simulink library "pack_105s34p_structured"  (R2023b)
settings: Solver=VariableStepAuto  StartTime=0.0  StopTime=10.0  RelTol=1e-3
undefined symbols (not defined in the file): battery_builder_rtmsupport, gcbh
libraries: pack_105s34p_structured_lib x156
(part 3 of 7)

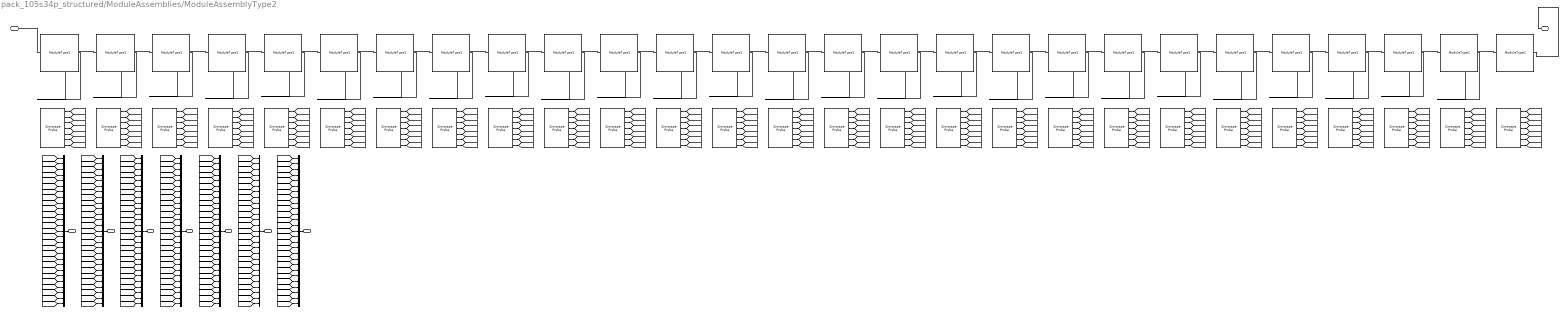
== system pack_105s34p_structured/ModuleAssemblies/ModuleAssemblyType2 ==
  note: Battery Modules
  note: Output Signals
  Module01 : pack_105s34p_structured_lib/Modules/ModuleType1  SOC_vecCell=[0, .1, .25, .5, .75, .9, 1]  T_vecCell=[278, 293, 313] K  V0_matCell=[3.49, 3.5, 3.51; 3.55, 3.57, 3.56; 3.62, 3.63, 3.64; 3.71, 3.71, 3.72; 3.91, 3.93, 3.94; 4.07, 4.08, 4.08; 4.19, 4.19, 4.19] V  V_rangeCell=[0, inf] V  R0_matCell=[.0117, .0085, .009; .011, .0085, .009; .0114, .0087, .0092; .0107, .0082, .0088; .0107, .0083, .0091; .0113, .0085, .0089; .0116, .0085, .0089] Ohm  AHCell=27 A*hr  extrapolation_optionCell=simscape.enum.extrapolation.nearest  R1_matCell=[.0109, .0029, .0013; .0069, .0024, .0012; .0047, .0026, .0013; .0034, .0016, .001; .0033, .0023, .0014; .0033, .0018, .0011; .0028, .0017, .0011] Ohm  tau1_matCell=[20, 36, 39; 31, 45, 39; 109, 105, 61; 36, 29, 26; 59, 77, 67; 40, 33, 29; 25, 39, 33] s  R2_matCell=[.0109, .0029, .0013; .0069, .0024, .0012; .0047, .0026, .0013; .0034, .0016, .001; .0033, .0023, .0014; .0033, .0018, .0011; .0028, .0017, .0011] Ohm  tau2_matCell=[20, 36, 39; 31, 45, 39; 109, 105, 61; 36, 29, 26; 59, 77, 67; 40, 33, 29; 25, 39, 33] s  R3_matCell=[.0109, .0029, .0013; .0069, .0024, .0012; .0047, .0026, .0013; .0034, .0016, .001; .0033, .0023, .0014; .0033, .0018, .0011; .0028, .0017, .0011] Ohm  tau3_matCell=[20, 36, 39; 31, 45, 39; 109, 105, 61; 36, 29, 26; 59, 77, 67; 40, 33, 29; 25, 39, 33] s  thermal_massCell=100 J/K  P=34  S=1  iCell_specify=off  iCell_priority=None  iCell=0 A  iCell_nominal_specify=off  iCell_nominal_unit=A  iCell_nominal_value=1  vCell_specify=off  vCell_priority=None  vCell=0 V  vCell_nominal_specify=off  vCell_nominal_unit=V  vCell_nominal_value=1  socCell_specify=off  socCell_priority=High  socCell=1  socCell_nominal_specify=off  socCell_nominal_unit=1  socCell_nominal_value=1  numCyclesCell_specify=off  numCyclesCell_priority=High  numCyclesCell=0  numCyclesCell_nominal_specify=off  numCyclesCell_nominal_unit=1  numCyclesCell_nominal_value=1  temperatureCell_specify=off  temperatureCell_priority=High  temperatureCell=298.15 K  temperatureCell_nominal_specify=off  temperatureCell_nominal_unit=K  temperatureCell_nominal_value=1  vParallelAssembly_specify=off  vParallelAssembly_priority=None  vParallelAssembly=0 V  vParallelAssembly_nominal_specify=off  vParallelAssembly_nominal_unit=V  vParallelAssembly_nominal_value=1  socParallelAssembly_specify=off  socParallelAssembly_priority=None  socParallelAssembly=1  socParallelAssembly_nominal_specify=off  socParallelAssembly_nominal_unit=1  socParallelAssembly_nominal_value=1
      settings: InternalSimscapePortConfiguration="{\"Bottom\":[{\"id\":\"n\",\"label\":\"-\",\"type\":\"foundation.electrical.electrical\"}],\"Left\":[],\"Right\":[],\"Top\":[{\"id\":\"p\",\"label\":\"+\",\"type\":\"foundation.electrical.electrical\"}]}"
  Module01_outputs : SimscapeProbe  BoundBlock=406  Variables={iCell, numCyclesCell, socCell, socParallelAssembly, temperatureCell, vCell, vParallelAssembly}
  Module02 : pack_105s34p_structured_lib/Modules/ModuleType1  SOC_vecCell=[0, .1, .25, .5, .75, .9, 1]  T_vecCell=[278, 293, 313] K  V0_matCell=[3.49, 3.5, 3.51; 3.55, 3.57, 3.56; 3.62, 3.63, 3.64; 3.71, 3.71, 3.72; 3.91, 3.93, 3.94; 4.07, 4.08, 4.08; 4.19, 4.19, 4.19] V  V_rangeCell=[0, inf] V  R0_matCell=[.0117, .0085, .009; .011, .0085, .009; .0114, .0087, .0092; .0107, .0082, .0088; .0107, .0083, .0091; .0113, .0085, .0089; .0116, .0085, .0089] Ohm  AHCell=27 A*hr  extrapolation_optionCell=simscape.enum.extrapolation.nearest  R1_matCell=[.0109, .0029, .0013; .0069, .0024, .0012; .0047, .0026, .0013; .0034, .0016, .001; .0033, .0023, .0014; .0033, .0018, .0011; .0028, .0017, .0011] Ohm  tau1_matCell=[20, 36, 39; 31, 45, 39; 109, 105, 61; 36, 29, 26; 59, 77, 67; 40, 33, 29; 25, 39, 33] s  R2_matCell=[.0109, .0029, .0013; .0069, .0024, .0012; .0047, .0026, .0013; .0034, .0016, .001; .0033, .0023, .0014; .0033, .0018, .0011; .0028, .0017, .0011] Ohm  tau2_matCell=[20, 36, 39; 31, 45, 39; 109, 105, 61; 36, 29, 26; 59, 77, 67; 40, 33, 29; 25, 39, 33] s  R3_matCell=[.0109, .0029, .0013; .0069, .0024, .0012; .0047, .0026, .0013; .0034, .0016, .001; .0033, .0023, .0014; .0033, .0018, .0011; .0028, .0017, .0011] Ohm  tau3_matCell=[20, 36, 39; 31, 45, 39; 109, 105, 61; 36, 29, 26; 59, 77, 67; 40, 33, 29; 25, 39, 33] s  thermal_massCell=100 J/K  P=34  S=1  iCell_specify=off  iCell_priority=None  iCell=0 A  iCell_nominal_specify=off  iCell_nominal_unit=A  iCell_nominal_value=1  vCell_specify=off  vCell_priority=None  vCell=0 V  vCell_nominal_specify=off  vCell_nominal_unit=V  vCell_nominal_value=1  socCell_specify=off  socCell_priority=High  socCell=1  socCell_nominal_specify=off  socCell_nominal_unit=1  socCell_nominal_value=1  numCyclesCell_specify=off  numCyclesCell_priority=High  numCyclesCell=0  numCyclesCell_nominal_specify=off  numCyclesCell_nominal_unit=1  numCyclesCell_nominal_value=1  temperatureCell_specify=off  temperatureCell_priority=High  temperatureCell=298.15 K  temperatureCell_nominal_specify=off  temperatureCell_nominal_unit=K  temperatureCell_nominal_value=1  vParallelAssembly_specify=off  vParallelAssembly_priority=None  vParallelAssembly=0 V  vParallelAssembly_nominal_specify=off  vParallelAssembly_nominal_unit=V  vParallelAssembly_nominal_value=1  socParallelAssembly_specify=off  socParallelAssembly_priority=None  socParallelAssembly=1  socParallelAssembly_nominal_specify=off  socParallelAssembly_nominal_unit=1  socParallelAssembly_nominal_value=1
      settings: InternalSimscapePortConfiguration="{\"Bottom\":[{\"id\":\"n\",\"label\":\"-\",\"type\":\"foundation.electrical.electrical\"}],\"Left\":[],\"Right\":[],\"Top\":[{\"id\":\"p\",\"label\":\"+\",\"type\":\"foundation.electrical.electrical\"}]}"
  Module02_outputs : SimscapeProbe  BoundBlock=407  Variables={iCell, numCyclesCell, socCell, socParallelAssembly, temperatureCell, vCell, vParallelAssembly}
  Module03 : pack_105s34p_structured_lib/Modules/ModuleType1  SOC_vecCell=[0, .1, .25, .5, .75, .9, 1]  T_vecCell=[278, 293, 313] K  V0_matCell=[3.49, 3.5, 3.51; 3.55, 3.57, 3.56; 3.62, 3.63, 3.64; 3.71, 3.71, 3.72; 3.91, 3.93, 3.94; 4.07, 4.08, 4.08; 4.19, 4.19, 4.19] V  V_rangeCell=[0, inf] V  R0_matCell=[.0117, .0085, .009; .011, .0085, .009; .0114, .0087, .0092; .0107, .0082, .0088; .0107, .0083, .0091; .0113, .0085, .0089; .0116, .0085, .0089] Ohm  AHCell=27 A*hr  extrapolation_optionCell=simscape.enum.extrapolation.nearest  R1_matCell=[.0109, .0029, .0013; .0069, .0024, .0012; .0047, .0026, .0013; .0034, .0016, .001; .0033, .0023, .0014; .0033, .0018, .0011; .0028, .0017, .0011] Ohm  tau1_matCell=[20, 36, 39; 31, 45, 39; 109, 105, 61; 36, 29, 26; 59, 77, 67; 40, 33, 29; 25, 39, 33] s  R2_matCell=[.0109, .0029, .0013; .0069, .0024, .0012; .0047, .0026, .0013; .0034, .0016, .001; .0033, .0023, .0014; .0033, .0018, .0011; .0028, .0017, .0011] Ohm  tau2_matCell=[20, 36, 39; 31, 45, 39; 109, 105, 61; 36, 29, 26; 59, 77, 67; 40, 33, 29; 25, 39, 33] s  R3_matCell=[.0109, .0029, .0013; .0069, .0024, .0012; .0047, .0026, .0013; .0034, .0016, .001; .0033, .0023, .0014; .0033, .0018, .0011; .0028, .0017, .0011] Ohm  tau3_matCell=[20, 36, 39; 31, 45, 39; 109, 105, 61; 36, 29, 26; 59, 77, 67; 40, 33, 29; 25, 39, 33] s  thermal_massCell=100 J/K  P=34  S=1  iCell_specify=off  iCell_priority=None  iCell=0 A  iCell_nominal_specify=off  iCell_nominal_unit=A  iCell_nominal_value=1  vCell_specify=off  vCell_priority=None  vCell=0 V  vCell_nominal_specify=off  vCell_nominal_unit=V  vCell_nominal_value=1  socCell_specify=off  socCell_priority=High  socCell=1  socCell_nominal_specify=off  socCell_nominal_unit=1  socCell_nominal_value=1  numCyclesCell_specify=off  numCyclesCell_priority=High  numCyclesCell=0  numCyclesCell_nominal_specify=off  numCyclesCell_nominal_unit=1  numCyclesCell_nominal_value=1  temperatureCell_specify=off  temperatureCell_priority=High  temperatureCell=298.15 K  temperatureCell_nominal_specify=off  temperatureCell_nominal_unit=K  temperatureCell_nominal_value=1  vParallelAssembly_specify=off  vParallelAssembly_priority=None  vParallelAssembly=0 V  vParallelAssembly_nominal_specify=off  vParallelAssembly_nominal_unit=V  vParallelAssembly_nominal_value=1  socParallelAssembly_specify=off  socParallelAssembly_priority=None  socParallelAssembly=1  socParallelAssembly_nominal_specify=off  socParallelAssembly_nominal_unit=1  socParallelAssembly_nominal_value=1
      settings: InternalSimscapePortConfiguration="{\"Bottom\":[{\"id\":\"n\",\"label\":\"-\",\"type\":\"foundation.electrical.electrical\"}],\"Left\":[],\"Right\":[],\"Top\":[{\"id\":\"p\",\"label\":\"+\",\"type\":\"foundation.electrical.electrical\"}]}"
  Module03_outputs : SimscapeProbe  BoundBlock=408  Variables={iCell, numCyclesCell, socCell, socParallelAssembly, temperatureCell, vCell, vParallelAssembly}
  Module04 : pack_105s34p_structured_lib/Modules/ModuleType1  SOC_vecCell=[0, .1, .25, .5, .75, .9, 1]  T_vecCell=[278, 293, 313] K  V0_matCell=[3.49, 3.5, 3.51; 3.55, 3.57, 3.56; 3.62, 3.63, 3.64; 3.71, 3.71, 3.72; 3.91, 3.93, 3.94; 4.07, 4.08, 4.08; 4.19, 4.19, 4.19] V  V_rangeCell=[0, inf] V  R0_matCell=[.0117, .0085, .009; .011, .0085, .009; .0114, .0087, .0092; .0107, .0082, .0088; .0107, .0083, .0091; .0113, .0085, .0089; .0116, .0085, .0089] Ohm  AHCell=27 A*hr  extrapolation_optionCell=simscape.enum.extrapolation.nearest  R1_matCell=[.0109, .0029, .0013; .0069, .0024, .0012; .0047, .0026, .0013; .0034, .0016, .001; .0033, .0023, .0014; .0033, .0018, .0011; .0028, .0017, .0011] Ohm  tau1_matCell=[20, 36, 39; 31, 45, 39; 109, 105, 61; 36, 29, 26; 59, 77, 67; 40, 33, 29; 25, 39, 33] s  R2_matCell=[.0109, .0029, .0013; .0069, .0024, .0012; .0047, .0026, .0013; .0034, .0016, .001; .0033, .0023, .0014; .0033, .0018, .0011; .0028, .0017, .0011] Ohm  tau2_matCell=[20, 36, 39; 31, 45, 39; 109, 105, 61; 36, 29, 26; 59, 77, 67; 40, 33, 29; 25, 39, 33] s  R3_matCell=[.0109, .0029, .0013; .0069, .0024, .0012; .0047, .0026, .0013; .0034, .0016, .001; .0033, .0023, .0014; .0033, .0018, .0011; .0028, .0017, .0011] Ohm  tau3_matCell=[20, 36, 39; 31, 45, 39; 109, 105, 61; 36, 29, 26; 59, 77, 67; 40, 33, 29; 25, 39, 33] s  thermal_massCell=100 J/K  P=34  S=1  iCell_specify=off  iCell_priority=None  iCell=0 A  iCell_nominal_specify=off  iCell_nominal_unit=A  iCell_nominal_value=1  vCell_specify=off  vCell_priority=None  vCell=0 V  vCell_nominal_specify=off  vCell_nominal_unit=V  vCell_nominal_value=1  socCell_specify=off  socCell_priority=High  socCell=1  socCell_nominal_specify=off  socCell_nominal_unit=1  socCell_nominal_value=1  numCyclesCell_specify=off  numCyclesCell_priority=High  numCyclesCell=0  numCyclesCell_nominal_specify=off  numCyclesCell_nominal_unit=1  numCyclesCell_nominal_value=1  temperatureCell_specify=off  temperatureCell_priority=High  temperatureCell=298.15 K  temperatureCell_nominal_specify=off  temperatureCell_nominal_unit=K  temperatureCell_nominal_value=1  vParallelAssembly_specify=off  vParallelAssembly_priority=None  vParallelAssembly=0 V  vParallelAssembly_nominal_specify=off  vParallelAssembly_nominal_unit=V  vParallelAssembly_nominal_value=1  socParallelAssembly_specify=off  socParallelAssembly_priority=None  socParallelAssembly=1  socParallelAssembly_nominal_specify=off  socParallelAssembly_nominal_unit=1  socParallelAssembly_nominal_value=1
      settings: InternalSimscapePortConfiguration="{\"Bottom\":[{\"id\":\"n\",\"label\":\"-\",\"type\":\"foundation.electrical.electrical\"}],\"Left\":[],\"Right\":[],\"Top\":[{\"id\":\"p\",\"label\":\"+\",\"type\":\"foundation.electrical.electrical\"}]}"
  Module04_outputs : SimscapeProbe  BoundBlock=409  Variables={iCell, numCyclesCell, socCell, socParallelAssembly, temperatureCell, vCell, vParallelAssembly}
  Module05 : pack_105s34p_structured_lib/Modules/ModuleType1  SOC_vecCell=[0, .1, .25, .5, .75, .9, 1]  T_vecCell=[278, 293, 313] K  V0_matCell=[3.49, 3.5, 3.51; 3.55, 3.57, 3.56; 3.62, 3.63, 3.64; 3.71, 3.71, 3.72; 3.91, 3.93, 3.94; 4.07, 4.08, 4.08; 4.19, 4.19, 4.19] V  V_rangeCell=[0, inf] V  R0_matCell=[.0117, .0085, .009; .011, .0085, .009; .0114, .0087, .0092; .0107, .0082, .0088; .0107, .0083, .0091; .0113, .0085, .0089; .0116, .0085, .0089] Ohm  AHCell=27 A*hr  extrapolation_optionCell=simscape.enum.extrapolation.nearest  R1_matCell=[.0109, .0029, .0013; .0069, .0024, .0012; .0047, .0026, .0013; .0034, .0016, .001; .0033, .0023, .0014; .0033, .0018, .0011; .0028, .0017, .0011] Ohm  tau1_matCell=[20, 36, 39; 31, 45, 39; 109, 105, 61; 36, 29, 26; 59, 77, 67; 40, 33, 29; 25, 39, 33] s  R2_matCell=[.0109, .0029, .0013; .0069, .0024, .0012; .0047, .0026, .0013; .0034, .0016, .001; .0033, .0023, .0014; .0033, .0018, .0011; .0028, .0017, .0011] Ohm  tau2_matCell=[20, 36, 39; 31, 45, 39; 109, 105, 61; 36, 29, 26; 59, 77, 67; 40, 33, 29; 25, 39, 33] s  R3_matCell=[.0109, .0029, .0013; .0069, .0024, .0012; .0047, .0026, .0013; .0034, .0016, .001; .0033, .0023, .0014; .0033, .0018, .0011; .0028, .0017, .0011] Ohm  tau3_matCell=[20, 36, 39; 31, 45, 39; 109, 105, 61; 36, 29, 26; 59, 77, 67; 40, 33, 29; 25, 39, 33] s  thermal_massCell=100 J/K  P=34  S=1  iCell_specify=off  iCell_priority=None  iCell=0 A  iCell_nominal_specify=off  iCell_nominal_unit=A  iCell_nominal_value=1  vCell_specify=off  vCell_priority=None  vCell=0 V  vCell_nominal_specify=off  vCell_nominal_unit=V  vCell_nominal_value=1  socCell_specify=off  socCell_priority=High  socCell=1  socCell_nominal_specify=off  socCell_nominal_unit=1  socCell_nominal_value=1  numCyclesCell_specify=off  numCyclesCell_priority=High  numCyclesCell=0  numCyclesCell_nominal_specify=off  numCyclesCell_nominal_unit=1  numCyclesCell_nominal_value=1  temperatureCell_specify=off  temperatureCell_priority=High  temperatureCell=298.15 K  temperatureCell_nominal_specify=off  temperatureCell_nominal_unit=K  temperatureCell_nominal_value=1  vParallelAssembly_specify=off  vParallelAssembly_priority=None  vParallelAssembly=0 V  vParallelAssembly_nominal_specify=off  vParallelAssembly_nominal_unit=V  vParallelAssembly_nominal_value=1  socParallelAssembly_specify=off  socParallelAssembly_priority=None  socParallelAssembly=1  socParallelAssembly_nominal_specify=off  socParallelAssembly_nominal_unit=1  socParallelAssembly_nominal_value=1
      settings: InternalSimscapePortConfiguration="{\"Bottom\":[{\"id\":\"n\",\"label\":\"-\",\"type\":\"foundation.electrical.electrical\"}],\"Left\":[],\"Right\":[],\"Top\":[{\"id\":\"p\",\"label\":\"+\",\"type\":\"foundation.electrical.electrical\"}]}"
  Module05_outputs : SimscapeProbe  BoundBlock=410  Variables={iCell, numCyclesCell, socCell, socParallelAssembly, temperatureCell, vCell, vParallelAssembly}
  Module06 : pack_105s34p_structured_lib/Modules/ModuleType1  SOC_vecCell=[0, .1, .25, .5, .75, .9, 1]  T_vecCell=[278, 293, 313] K  V0_matCell=[3.49, 3.5, 3.51; 3.55, 3.57, 3.56; 3.62, 3.63, 3.64; 3.71, 3.71, 3.72; 3.91, 3.93, 3.94; 4.07, 4.08, 4.08; 4.19, 4.19, 4.19] V  V_rangeCell=[0, inf] V  R0_matCell=[.0117, .0085, .009; .011, .0085, .009; .0114, .0087, .0092; .0107, .0082, .0088; .0107, .0083, .0091; .0113, .0085, .0089; .0116, .0085, .0089] Ohm  AHCell=27 A*hr  extrapolation_optionCell=simscape.enum.extrapolation.nearest  R1_matCell=[.0109, .0029, .0013; .0069, .0024, .0012; .0047, .0026, .0013; .0034, .0016, .001; .0033, .0023, .0014; .0033, .0018, .0011; .0028, .0017, .0011] Ohm  tau1_matCell=[20, 36, 39; 31, 45, 39; 109, 105, 61; 36, 29, 26; 59, 77, 67; 40, 33, 29; 25, 39, 33] s  R2_matCell=[.0109, .0029, .0013; .0069, .0024, .0012; .0047, .0026, .0013; .0034, .0016, .001; .0033, .0023, .0014; .0033, .0018, .0011; .0028, .0017, .0011] Ohm  tau2_matCell=[20, 36, 39; 31, 45, 39; 109, 105, 61; 36, 29, 26; 59, 77, 67; 40, 33, 29; 25, 39, 33] s  R3_matCell=[.0109, .0029, .0013; .0069, .0024, .0012; .0047, .0026, .0013; .0034, .0016, .001; .0033, .0023, .0014; .0033, .0018, .0011; .0028, .0017, .0011] Ohm  tau3_matCell=[20, 36, 39; 31, 45, 39; 109, 105, 61; 36, 29, 26; 59, 77, 67; 40, 33, 29; 25, 39, 33] s  thermal_massCell=100 J/K  P=34  S=1  iCell_specify=off  iCell_priority=None  iCell=0 A  iCell_nominal_specify=off  iCell_nominal_unit=A  iCell_nominal_value=1  vCell_specify=off  vCell_priority=None  vCell=0 V  vCell_nominal_specify=off  vCell_nominal_unit=V  vCell_nominal_value=1  socCell_specify=off  socCell_priority=High  socCell=1  socCell_nominal_specify=off  socCell_nominal_unit=1  socCell_nominal_value=1  numCyclesCell_specify=off  numCyclesCell_priority=High  numCyclesCell=0  numCyclesCell_nominal_specify=off  numCyclesCell_nominal_unit=1  numCyclesCell_nominal_value=1  temperatureCell_specify=off  temperatureCell_priority=High  temperatureCell=298.15 K  temperatureCell_nominal_specify=off  temperatureCell_nominal_unit=K  temperatureCell_nominal_value=1  vParallelAssembly_specify=off  vParallelAssembly_priority=None  vParallelAssembly=0 V  vParallelAssembly_nominal_specify=off  vParallelAssembly_nominal_unit=V  vParallelAssembly_nominal_value=1  socParallelAssembly_specify=off  socParallelAssembly_priority=None  socParallelAssembly=1  socParallelAssembly_nominal_specify=off  socParallelAssembly_nominal_unit=1  socParallelAssembly_nominal_value=1
      settings: InternalSimscapePortConfiguration="{\"Bottom\":[{\"id\":\"n\",\"label\":\"-\",\"type\":\"foundation.electrical.electrical\"}],\"Left\":[],\"Right\":[],\"Top\":[{\"id\":\"p\",\"label\":\"+\",\"type\":\"foundation.electrical.electrical\"}]}"
  Module06_outputs : SimscapeProbe  BoundBlock=411  Variables={iCell, numCyclesCell, socCell, socParallelAssembly, temperatureCell, vCell, vParallelAssembly}
  Module07 : pack_105s34p_structured_lib/Modules/ModuleType1  SOC_vecCell=[0, .1, .25, .5, .75, .9, 1]  T_vecCell=[278, 293, 313] K  V0_matCell=[3.49, 3.5, 3.51; 3.55, 3.57, 3.56; 3.62, 3.63, 3.64; 3.71, 3.71, 3.72; 3.91, 3.93, 3.94; 4.07, 4.08, 4.08; 4.19, 4.19, 4.19] V  V_rangeCell=[0, inf] V  R0_matCell=[.0117, .0085, .009; .011, .0085, .009; .0114, .0087, .0092; .0107, .0082, .0088; .0107, .0083, .0091; .0113, .0085, .0089; .0116, .0085, .0089] Ohm  AHCell=27 A*hr  extrapolation_optionCell=simscape.enum.extrapolation.nearest  R1_matCell=[.0109, .0029, .0013; .0069, .0024, .0012; .0047, .0026, .0013; .0034, .0016, .001; .0033, .0023, .0014; .0033, .0018, .0011; .0028, .0017, .0011] Ohm  tau1_matCell=[20, 36, 39; 31, 45, 39; 109, 105, 61; 36, 29, 26; 59, 77, 67; 40, 33, 29; 25, 39, 33] s  R2_matCell=[.0109, .0029, .0013; .0069, .0024, .0012; .0047, .0026, .0013; .0034, .0016, .001; .0033, .0023, .0014; .0033, .0018, .0011; .0028, .0017, .0011] Ohm  tau2_matCell=[20, 36, 39; 31, 45, 39; 109, 105, 61; 36, 29, 26; 59, 77, 67; 40, 33, 29; 25, 39, 33] s  R3_matCell=[.0109, .0029, .0013; .0069, .0024, .0012; .0047, .0026, .0013; .0034, .0016, .001; .0033, .0023, .0014; .0033, .0018, .0011; .0028, .0017, .0011] Ohm  tau3_matCell=[20, 36, 39; 31, 45, 39; 109, 105, 61; 36, 29, 26; 59, 77, 67; 40, 33, 29; 25, 39, 33] s  thermal_massCell=100 J/K  P=34  S=1  iCell_specify=off  iCell_priority=None  iCell=0 A  iCell_nominal_specify=off  iCell_nominal_unit=A  iCell_nominal_value=1  vCell_specify=off  vCell_priority=None  vCell=0 V  vCell_nominal_specify=off  vCell_nominal_unit=V  vCell_nominal_value=1  socCell_specify=off  socCell_priority=High  socCell=1  socCell_nominal_specify=off  socCell_nominal_unit=1  socCell_nominal_value=1  numCyclesCell_specify=off  numCyclesCell_priority=High  numCyclesCell=0  numCyclesCell_nominal_specify=off  numCyclesCell_nominal_unit=1  numCyclesCell_nominal_value=1  temperatureCell_specify=off  temperatureCell_priority=High  temperatureCell=298.15 K  temperatureCell_nominal_specify=off  temperatureCell_nominal_unit=K  temperatureCell_nominal_value=1  vParallelAssembly_specify=off  vParallelAssembly_priority=None  vParallelAssembly=0 V  vParallelAssembly_nominal_specify=off  vParallelAssembly_nominal_unit=V  vParallelAssembly_nominal_value=1  socParallelAssembly_specify=off  socParallelAssembly_priority=None  socParallelAssembly=1  socParallelAssembly_nominal_specify=off  socParallelAssembly_nominal_unit=1  socParallelAssembly_nominal_value=1
      settings: InternalSimscapePortConfiguration="{\"Bottom\":[{\"id\":\"n\",\"label\":\"-\",\"type\":\"foundation.electrical.electrical\"}],\"Left\":[],\"Right\":[],\"Top\":[{\"id\":\"p\",\"label\":\"+\",\"type\":\"foundation.electrical.electrical\"}]}"
  Module07_outputs : SimscapeProbe  BoundBlock=412  Variables={iCell, numCyclesCell, socCell, socParallelAssembly, temperatureCell, vCell, vParallelAssembly}
  Module08 : pack_105s34p_structured_lib/Modules/ModuleType1  SOC_vecCell=[0, .1, .25, .5, .75, .9, 1]  T_vecCell=[278, 293, 313] K  V0_matCell=[3.49, 3.5, 3.51; 3.55, 3.57, 3.56; 3.62, 3.63, 3.64; 3.71, 3.71, 3.72; 3.91, 3.93, 3.94; 4.07, 4.08, 4.08; 4.19, 4.19, 4.19] V  V_rangeCell=[0, inf] V  R0_matCell=[.0117, .0085, .009; .011, .0085, .009; .0114, .0087, .0092; .0107, .0082, .0088; .0107, .0083, .0091; .0113, .0085, .0089; .0116, .0085, .0089] Ohm  AHCell=27 A*hr  extrapolation_optionCell=simscape.enum.extrapolation.nearest  R1_matCell=[.0109, .0029, .0013; .0069, .0024, .0012; .0047, .0026, .0013; .0034, .0016, .001; .0033, .0023, .0014; .0033, .0018, .0011; .0028, .0017, .0011] Ohm  tau1_matCell=[20, 36, 39; 31, 45, 39; 109, 105, 61; 36, 29, 26; 59, 77, 67; 40, 33, 29; 25, 39, 33] s  R2_matCell=[.0109, .0029, .0013; .0069, .0024, .0012; .0047, .0026, .0013; .0034, .0016, .001; .0033, .0023, .0014; .0033, .0018, .0011; .0028, .0017, .0011] Ohm  tau2_matCell=[20, 36, 39; 31, 45, 39; 109, 105, 61; 36, 29, 26; 59, 77, 67; 40, 33, 29; 25, 39, 33] s  R3_matCell=[.0109, .0029, .0013; .0069, .0024, .0012; .0047, .0026, .0013; .0034, .0016, .001; .0033, .0023, .0014; .0033, .0018, .0011; .0028, .0017, .0011] Ohm  tau3_matCell=[20, 36, 39; 31, 45, 39; 109, 105, 61; 36, 29, 26; 59, 77, 67; 40, 33, 29; 25, 39, 33] s  thermal_massCell=100 J/K  P=34  S=1  iCell_specify=off  iCell_priority=None  iCell=0 A  iCell_nominal_specify=off  iCell_nominal_unit=A  iCell_nominal_value=1  vCell_specify=off  vCell_priority=None  vCell=0 V  vCell_nominal_specify=off  vCell_nominal_unit=V  vCell_nominal_value=1  socCell_specify=off  socCell_priority=High  socCell=1  socCell_nominal_specify=off  socCell_nominal_unit=1  socCell_nominal_value=1  numCyclesCell_specify=off  numCyclesCell_priority=High  numCyclesCell=0  numCyclesCell_nominal_specify=off  numCyclesCell_nominal_unit=1  numCyclesCell_nominal_value=1  temperatureCell_specify=off  temperatureCell_priority=High  temperatureCell=298.15 K  temperatureCell_nominal_specify=off  temperatureCell_nominal_unit=K  temperatureCell_nominal_value=1  vParallelAssembly_specify=off  vParallelAssembly_priority=None  vParallelAssembly=0 V  vParallelAssembly_nominal_specify=off  vParallelAssembly_nominal_unit=V  vParallelAssembly_nominal_value=1  socParallelAssembly_specify=off  socParallelAssembly_priority=None  socParallelAssembly=1  socParallelAssembly_nominal_specify=off  socParallelAssembly_nominal_unit=1  socParallelAssembly_nominal_value=1
      settings: InternalSimscapePortConfiguration="{\"Bottom\":[{\"id\":\"n\",\"label\":\"-\",\"type\":\"foundation.electrical.electrical\"}],\"Left\":[],\"Right\":[],\"Top\":[{\"id\":\"p\",\"label\":\"+\",\"type\":\"foundation.electrical.electrical\"}]}"
  Module08_outputs : SimscapeProbe  BoundBlock=413  Variables={iCell, numCyclesCell, socCell, socParallelAssembly, temperatureCell, vCell, vParallelAssembly}
  Module09 : pack_105s34p_structured_lib/Modules/ModuleType1  SOC_vecCell=[0, .1, .25, .5, .75, .9, 1]  T_vecCell=[278, 293, 313] K  V0_matCell=[3.49, 3.5, 3.51; 3.55, 3.57, 3.56; 3.62, 3.63, 3.64; 3.71, 3.71, 3.72; 3.91, 3.93, 3.94; 4.07, 4.08, 4.08; 4.19, 4.19, 4.19] V  V_rangeCell=[0, inf] V  R0_matCell=[.0117, .0085, .009; .011, .0085, .009; .0114, .0087, .0092; .0107, .0082, .0088; .0107, .0083, .0091; .0113, .0085, .0089; .0116, .0085, .0089] Ohm  AHCell=27 A*hr  extrapolation_optionCell=simscape.enum.extrapolation.nearest  R1_matCell=[.0109, .0029, .0013; .0069, .0024, .0012; .0047, .0026, .0013; .0034, .0016, .001; .0033, .0023, .0014; .0033, .0018, .0011; .0028, .0017, .0011] Ohm  tau1_matCell=[20, 36, 39; 31, 45, 39; 109, 105, 61; 36, 29, 26; 59, 77, 67; 40, 33, 29; 25, 39, 33] s  R2_matCell=[.0109, .0029, .0013; .0069, .0024, .0012; .0047, .0026, .0013; .0034, .0016, .001; .0033, .0023, .0014; .0033, .0018, .0011; .0028, .0017, .0011] Ohm  tau2_matCell=[20, 36, 39; 31, 45, 39; 109, 105, 61; 36, 29, 26; 59, 77, 67; 40, 33, 29; 25, 39, 33] s  R3_matCell=[.0109, .0029, .0013; .0069, .0024, .0012; .0047, .0026, .0013; .0034, .0016, .001; .0033, .0023, .0014; .0033, .0018, .0011; .0028, .0017, .0011] Ohm  tau3_matCell=[20, 36, 39; 31, 45, 39; 109, 105, 61; 36, 29, 26; 59, 77, 67; 40, 33, 29; 25, 39, 33] s  thermal_massCell=100 J/K  P=34  S=1  iCell_specify=off  iCell_priority=None  iCell=0 A  iCell_nominal_specify=off  iCell_nominal_unit=A  iCell_nominal_value=1  vCell_specify=off  vCell_priority=None  vCell=0 V  vCell_nominal_specify=off  vCell_nominal_unit=V  vCell_nominal_value=1  socCell_specify=off  socCell_priority=High  socCell=1  socCell_nominal_specify=off  socCell_nominal_unit=1  socCell_nominal_value=1  numCyclesCell_specify=off  numCyclesCell_priority=High  numCyclesCell=0  numCyclesCell_nominal_specify=off  numCyclesCell_nominal_unit=1  numCyclesCell_nominal_value=1  temperatureCell_specify=off  temperatureCell_priority=High  temperatureCell=298.15 K  temperatureCell_nominal_specify=off  temperatureCell_nominal_unit=K  temperatureCell_nominal_value=1  vParallelAssembly_specify=off  vParallelAssembly_priority=None  vParallelAssembly=0 V  vParallelAssembly_nominal_specify=off  vParallelAssembly_nominal_unit=V  vParallelAssembly_nominal_value=1  socParallelAssembly_specify=off  socParallelAssembly_priority=None  socParallelAssembly=1  socParallelAssembly_nominal_specify=off  socParallelAssembly_nominal_unit=1  socParallelAssembly_nominal_value=1
      settings: InternalSimscapePortConfiguration="{\"Bottom\":[{\"id\":\"n\",\"label\":\"-\",\"type\":\"foundation.electrical.electrical\"}],\"Left\":[],\"Right\":[],\"Top\":[{\"id\":\"p\",\"label\":\"+\",\"type\":\"foundation.electrical.electrical\"}]}"
  Module09_outputs : SimscapeProbe  BoundBlock=414  Variables={iCell, numCyclesCell, socCell, socParallelAssembly, temperatureCell, vCell, vParallelAssembly}
  Module{10..27} (18 alike) : pack_105s34p_structured_lib/Modules/ModuleType1  SOC_vecCell=[0, .1, .25, .5, .75, .9, 1]  T_vecCell=[278, 293, 313] K  V0_matCell=[3.49, 3.5, 3.51; 3.55, 3.57, 3.56; 3.62, 3.63, 3.64; 3.71, 3.71, 3.72; 3.91, 3.93, 3.94; 4.07, 4.08, 4.08; 4.19, 4.19, 4.19] V  V_rangeCell=[0, inf] V  R0_matCell=[.0117, .0085, .009; .011, .0085, .009; .0114, .0087, .0092; .0107, .0082, .0088; .0107, .0083, .0091; .0113, .0085, .0089; .0116, .0085, .0089] Ohm  AHCell=27 A*hr  extrapolation_optionCell=simscape.enum.extrapolation.nearest  R1_matCell=[.0109, .0029, .0013; .0069, .0024, .0012; .0047, .0026, .0013; .0034, .0016, .001; .0033, .0023, .0014; .0033, .0018, .0011; .0028, .0017, .0011] Ohm  tau1_matCell=[20, 36, 39; 31, 45, 39; 109, 105, 61; 36, 29, 26; 59, 77, 67; 40, 33, 29; 25, 39, 33] s  R2_matCell=[.0109, .0029, .0013; .0069, .0024, .0012; .0047, .0026, .0013; .0034, .0016, .001; .0033, .0023, .0014; .0033, .0018, .0011; .0028, .0017, .0011] Ohm  tau2_matCell=[20, 36, 39; 31, 45, 39; 109, 105, 61; 36, 29, 26; 59, 77, 67; 40, 33, 29; 25, 39, 33] s  R3_matCell=[.0109, .0029, .0013; .0069, .0024, .0012; .0047, .0026, .0013; .0034, .0016, .001; .0033, .0023, .0014; .0033, .0018, .0011; .0028, .0017, .0011] Ohm  tau3_matCell=[20, 36, 39; 31, 45, 39; 109, 105, 61; 36, 29, 26; 59, 77, 67; 40, 33, 29; 25, 39, 33] s  thermal_massCell=100 J/K  P=34  S=1  iCell_specify=off  iCell_priority=None  iCell=0 A  iCell_nominal_specify=off  iCell_nominal_unit=A  iCell_nominal_value=1  vCell_specify=off  vCell_priority=None  vCell=0 V  vCell_nominal_specify=off  vCell_nominal_unit=V  vCell_nominal_value=1  socCell_specify=off  socCell_priority=High  socCell=1  socCell_nominal_specify=off  socCell_nominal_unit=1  socCell_nominal_value=1  numCyclesCell_specify=off  numCyclesCell_priority=High  numCyclesCell=0  numCyclesCell_nominal_specify=off  numCyclesCell_nominal_unit=1  numCyclesCell_nominal_value=1  temperatureCell_specify=off  temperatureCell_priority=High  temperatureCell=298.15 K  temperatureCell_nominal_specify=off  temperatureCell_nominal_unit=K  temperatureCell_nominal_value=1  vParallelAssembly_specify=off  vParallelAssembly_priority=None  vParallelAssembly=0 V  vParallelAssembly_nominal_specify=off  vParallelAssembly_nominal_unit=V  vParallelAssembly_nominal_value=1  socParallelAssembly_specify=off  socParallelAssembly_priority=None  socParallelAssembly=1  socParallelAssembly_nominal_specify=off  socParallelAssembly_nominal_unit=1  socParallelAssembly_nominal_value=1
      settings: InternalSimscapePortConfiguration="{\"Bottom\":[{\"id\":\"n\",\"label\":\"-\",\"type\":\"foundation.electrical.electrical\"}],\"Left\":[],\"Right\":[],\"Top\":[{\"id\":\"p\",\"label\":\"+\",\"type\":\"foundation.electrical.electrical\"}]}"
  Module10_outputs : SimscapeProbe  BoundBlock=415  Variables={iCell, numCyclesCell, socCell, socParallelAssembly, temperatureCell, vCell, vParallelAssembly}
  Module11_outputs : SimscapeProbe  BoundBlock=416  Variables={iCell, numCyclesCell, socCell, socParallelAssembly, temperatureCell, vCell, vParallelAssembly}
  Module12_outputs : SimscapeProbe  BoundBlock=417  Variables={iCell, numCyclesCell, socCell, socParallelAssembly, temperatureCell, vCell, vParallelAssembly}
  Module13_outputs : SimscapeProbe  BoundBlock=418  Variables={iCell, numCyclesCell, socCell, socParallelAssembly, temperatureCell, vCell, vParallelAssembly}
  Module14_outputs : SimscapeProbe  BoundBlock=419  Variables={iCell, numCyclesCell, socCell, socParallelAssembly, temperatureCell, vCell, vParallelAssembly}
  Module15_outputs : SimscapeProbe  BoundBlock=420  Variables={iCell, numCyclesCell, socCell, socParallelAssembly, temperatureCell, vCell, vParallelAssembly}
  Module16_outputs : SimscapeProbe  BoundBlock=421  Variables={iCell, numCyclesCell, socCell, socParallelAssembly, temperatureCell, vCell, vParallelAssembly}
  Module17_outputs : SimscapeProbe  BoundBlock=422  Variables={iCell, numCyclesCell, socCell, socParallelAssembly, temperatureCell, vCell, vParallelAssembly}
  Module18_outputs : SimscapeProbe  BoundBlock=423  Variables={iCell, numCyclesCell, socCell, socParallelAssembly, temperatureCell, vCell, vParallelAssembly}
  Module19_outputs : SimscapeProbe  BoundBlock=424  Variables={iCell, numCyclesCell, socCell, socParallelAssembly, temperatureCell, vCell, vParallelAssembly}
  Module20_outputs : SimscapeProbe  BoundBlock=425  Variables={iCell, numCyclesCell, socCell, socParallelAssembly, temperatureCell, vCell, vParallelAssembly}
  Module21_outputs : SimscapeProbe  BoundBlock=426  Variables={iCell, numCyclesCell, socCell, socParallelAssembly, temperatureCell, vCell, vParallelAssembly}
  Module22_outputs : SimscapeProbe  BoundBlock=427  Variables={iCell, numCyclesCell, socCell, socParallelAssembly, temperatureCell, vCell, vParallelAssembly}
  Module23_outputs : SimscapeProbe  BoundBlock=428  Variables={iCell, numCyclesCell, socCell, socParallelAssembly, temperatureCell, vCell, vParallelAssembly}
  Module24_outputs : SimscapeProbe  BoundBlock=429  Variables={iCell, numCyclesCell, socCell, socParallelAssembly, temperatureCell, vCell, vParallelAssembly}
  Module25_outputs : SimscapeProbe  BoundBlock=430  Variables={iCell, numCyclesCell, socCell, socParallelAssembly, temperatureCell, vCell, vParallelAssembly}
  Module26_outputs : SimscapeProbe  BoundBlock=431  Variables={iCell, numCyclesCell, socCell, socParallelAssembly, temperatureCell, vCell, vParallelAssembly}
  Module27_outputs : SimscapeProbe  BoundBlock=432  Variables={iCell, numCyclesCell, socCell, socParallelAssembly, temperatureCell, vCell, vParallelAssembly}
  iCellMux : Mux  Inputs=27
  numCyclesCellMux : Mux  Inputs=27
  socCellMux : Mux  Inputs=27
  socParallelAssemblyMux : Mux  Inputs=27
  temperatureCellMux : Mux  Inputs=27
  vCellMux : Mux  Inputs=27
  vParallelAssemblyMux : Mux  Inputs=27
  + : PMIOPort  Side=Left
  - : PMIOPort  Port=2  Side=Right
  iCell : Outport
  numCyclesCell : Outport  Port=2
  socCell : Outport  Port=3
  socParallelAssembly : Outport  Port=4
  temperatureCell : Outport  Port=5
  vCell : Outport  Port=6
  vParallelAssembly : Outport  Port=7
  wires:
  Module01_outputs/1 -> [iCell1]
  iCellMux/1 -> iCell/1
  [iCell1] -> iCellMux/1
  Module01_outputs/2 -> [numCyclesCell1]
  numCyclesCellMux/1 -> numCyclesCell/1
  [numCyclesCell1] -> numCyclesCellMux/1
  Module01_outputs/3 -> [socCell1]
  socCellMux/1 -> socCell/1
  [socCell1] -> socCellMux/1
  Module01_outputs/4 -> [socParallelAssembly1]
  socParallelAssemblyMux/1 -> socParallelAssembly/1
  [socParallelAssembly1] -> socParallelAssemblyMux/1
  Module01_outputs/5 -> [temperatureCell1]
  temperatureCellMux/1 -> temperatureCell/1
  [temperatureCell1] -> temperatureCellMux/1
  Module01_outputs/6 -> [vCell1]
  vCellMux/1 -> vCell/1
  [vCell1] -> vCellMux/1
  Module01_outputs/7 -> [vParallelAssembly1]
  vParallelAssemblyMux/1 -> vParallelAssembly/1
  [vParallelAssembly1] -> vParallelAssemblyMux/1
  Module02_outputs/1 -> [iCell2]
  [iCell2] -> iCellMux/2
  Module02_outputs/2 -> [numCyclesCell2]
  [numCyclesCell2] -> numCyclesCellMux/2
  Module02_outputs/3 -> [socCell2]
  [socCell2] -> socCellMux/2
  Module02_outputs/4 -> [socParallelAssembly2]
  [socParallelAssembly2] -> socParallelAssemblyMux/2
  Module02_outputs/5 -> [temperatureCell2]
  [temperatureCell2] -> temperatureCellMux/2
  Module02_outputs/6 -> [vCell2]
  [vCell2] -> vCellMux/2
  Module02_outputs/7 -> [vParallelAssembly2]
  [vParallelAssembly2] -> vParallelAssemblyMux/2
  Module03_outputs/1 -> [iCell3]
  [iCell3] -> iCellMux/3
  Module03_outputs/2 -> [numCyclesCell3]
  [numCyclesCell3] -> numCyclesCellMux/3
  Module03_outputs/3 -> [socCell3]
  [socCell3] -> socCellMux/3
  Module03_outputs/4 -> [socParallelAssembly3]
  [socParallelAssembly3] -> socParallelAssemblyMux/3
  Module03_outputs/5 -> [temperatureCell3]
  [temperatureCell3] -> temperatureCellMux/3
  Module03_outputs/6 -> [vCell3]
  [vCell3] -> vCellMux/3
  Module03_outputs/7 -> [vParallelAssembly3]
  [vParallelAssembly3] -> vParallelAssemblyMux/3
  Module04_outputs/1 -> [iCell4]
  [iCell4] -> iCellMux/4
  Module04_outputs/2 -> [numCyclesCell4]
  [numCyclesCell4] -> numCyclesCellMux/4
  Module04_outputs/3 -> [socCell4]
  [socCell4] -> socCellMux/4
  Module04_outputs/4 -> [socParallelAssembly4]
  [socParallelAssembly4] -> socParallelAssemblyMux/4
  Module04_outputs/5 -> [temperatureCell4]
  [temperatureCell4] -> temperatureCellMux/4
  Module04_outputs/6 -> [vCell4]
  [vCell4] -> vCellMux/4
  Module04_outputs/7 -> [vParallelAssembly4]
  [vParallelAssembly4] -> vParallelAssemblyMux/4
  Module05_outputs/1 -> [iCell5]
  [iCell5] -> iCellMux/5
  Module05_outputs/2 -> [numCyclesCell5]
  [numCyclesCell5] -> numCyclesCellMux/5
  Module05_outputs/3 -> [socCell5]
  [socCell5] -> socCellMux/5
  Module05_outputs/4 -> [socParallelAssembly5]
  [socParallelAssembly5] -> socParallelAssemblyMux/5
  Module05_outputs/5 -> [temperatureCell5]
  [temperatureCell5] -> temperatureCellMux/5
  Module05_outputs/6 -> [vCell5]
  [vCell5] -> vCellMux/5
  Module05_outputs/7 -> [vParallelAssembly5]
  [vParallelAssembly5] -> vParallelAssemblyMux/5
  Module06_outputs/1 -> [iCell6]
  [iCell6] -> iCellMux/6
  Module06_outputs/2 -> [numCyclesCell6]
  [numCyclesCell6] -> numCyclesCellMux/6
  Module06_outputs/3 -> [socCell6]
  [socCell6] -> socCellMux/6
  Module06_outputs/4 -> [socParallelAssembly6]
  [socParallelAssembly6] -> socParallelAssemblyMux/6
  Module06_outputs/5 -> [temperatureCell6]
  [temperatureCell6] -> temperatureCellMux/6
  Module06_outputs/6 -> [vCell6]
  [vCell6] -> vCellMux/6
  Module06_outputs/7 -> [vParallelAssembly6]
  [vParallelAssembly6] -> vParallelAssemblyMux/6
  Module07_outputs/1 -> [iCell7]
  [iCell7] -> iCellMux/7
  Module07_outputs/2 -> [numCyclesCell7]
  [numCyclesCell7] -> numCyclesCellMux/7
  Module07_outputs/3 -> [socCell7]
  [socCell7] -> socCellMux/7
  Module07_outputs/4 -> [socParallelAssembly7]
  [socParallelAssembly7] -> socParallelAssemblyMux/7
  Module07_outputs/5 -> [temperatureCell7]
  [temperatureCell7] -> temperatureCellMux/7
  Module07_outputs/6 -> [vCell7]
  [vCell7] -> vCellMux/7
  Module07_outputs/7 -> [vParallelAssembly7]
  [vParallelAssembly7] -> vParallelAssemblyMux/7
  Module08_outputs/1 -> [iCell8]
  [iCell8] -> iCellMux/8
  Module08_outputs/2 -> [numCyclesCell8]
  [numCyclesCell8] -> numCyclesCellMux/8
  Module08_outputs/3 -> [socCell8]
  [socCell8] -> socCellMux/8
  Module08_outputs/4 -> [socParallelAssembly8]
  [socParallelAssembly8] -> socParallelAssemblyMux/8
  Module08_outputs/5 -> [temperatureCell8]
  [temperatureCell8] -> temperatureCellMux/8
  Module08_outputs/6 -> [vCell8]
  [vCell8] -> vCellMux/8
  Module08_outputs/7 -> [vParallelAssembly8]
  [vParallelAssembly8] -> vParallelAssemblyMux/8
  Module09_outputs/1 -> [iCell9]
  [iCell9] -> iCellMux/9
  Module09_outputs/2 -> [numCyclesCell9]
  [numCyclesCell9] -> numCyclesCellMux/9
  Module09_outputs/3 -> [socCell9]
  [socCell9] -> socCellMux/9
  Module09_outputs/4 -> [socParallelAssembly9]
  [socParallelAssembly9] -> socParallelAssemblyMux/9
  Module09_outputs/5 -> [temperatureCell9]
  [temperatureCell9] -> temperatureCellMux/9
  Module09_outputs/6 -> [vCell9]
  [vCell9] -> vCellMux/9
  Module09_outputs/7 -> [vParallelAssembly9]
  [vParallelAssembly9] -> vParallelAssemblyMux/9
  Module10_outputs/1 -> [iCell10]
  [iCell10] -> iCellMux/10
  Module10_outputs/2 -> [numCyclesCell10]
  [numCyclesCell10] -> numCyclesCellMux/10
  Module10_outputs/3 -> [socCell10]
  [socCell10] -> socCellMux/10
  Module10_outputs/4 -> [socParallelAssembly10]
  [socParallelAssembly10] -> socParallelAssemblyMux/10
  Module10_outputs/5 -> [temperatureCell10]
  [temperatureCell10] -> temperatureCellMux/10
  Module10_outputs/6 -> [vCell10]
  [vCell10] -> vCellMux/10
  Module10_outputs/7 -> [vParallelAssembly10]
  [vParallelAssembly10] -> vParallelAssemblyMux/10
  Module11_outputs/1 -> [iCell11]
  [iCell11] -> iCellMux/11
  Module11_outputs/2 -> [numCyclesCell11]
  [numCyclesCell11] -> numCyclesCellMux/11
  Module11_outputs/3 -> [socCell11]
  [socCell11] -> socCellMux/11
  Module11_outputs/4 -> [socParallelAssembly11]
  [socParallelAssembly11] -> socParallelAssemblyMux/11
  Module11_outputs/5 -> [temperatureCell11]
  [temperatureCell11] -> temperatureCellMux/11
  Module11_outputs/6 -> [vCell11]
  [vCell11] -> vCellMux/11
  Module11_outputs/7 -> [vParallelAssembly11]
  [vParallelAssembly11] -> vParallelAssemblyMux/11
  Module12_outputs/1 -> [iCell12]
  [iCell12] -> iCellMux/12
  Module12_outputs/2 -> [numCyclesCell12]
  [numCyclesCell12] -> numCyclesCellMux/12
  Module12_outputs/3 -> [socCell12]
  [socCell12] -> socCellMux/12
  Module12_outputs/4 -> [socParallelAssembly12]
  [socParallelAssembly12] -> socParallelAssemblyMux/12
  Module12_outputs/5 -> [temperatureCell12]
  [temperatureCell12] -> temperatureCellMux/12
  Module12_outputs/6 -> [vCell12]
  [vCell12] -> vCellMux/12
  Module12_outputs/7 -> [vParallelAssembly12]
  [vParallelAssembly12] -> vParallelAssemblyMux/12
  Module13_outputs/1 -> [iCell13]
  [iCell13] -> iCellMux/13
  Module13_outputs/2 -> [numCyclesCell13]
  [numCyclesCell13] -> numCyclesCellMux/13
  Module13_outputs/3 -> [socCell13]
  [socCell13] -> socCellMux/13
  Module13_outputs/4 -> [socParallelAssembly13]
  [socParallelAssembly13] -> socParallelAssemblyMux/13
  Module13_outputs/5 -> [temperatureCell13]
  [temperatureCell13] -> temperatureCellMux/13
  Module13_outputs/6 -> [vCell13]
  [vCell13] -> vCellMux/13
  Module13_outputs/7 -> [vParallelAssembly13]
  [vParallelAssembly13] -> vParallelAssemblyMux/13
  Module14_outputs/1 -> [iCell14]
  [iCell14] -> iCellMux/14
  Module14_outputs/2 -> [numCyclesCell14]
  [numCyclesCell14] -> numCyclesCellMux/14
  Module14_outputs/3 -> [socCell14]
  [socCell14] -> socCellMux/14
  Module14_outputs/4 -> [socParallelAssembly14]
  [socParallelAssembly14] -> socParallelAssemblyMux/14
  Module14_outputs/5 -> [temperatureCell14]
  [temperatureCell14] -> temperatureCellMux/14
  Module14_outputs/6 -> [vCell14]
  [vCell14] -> vCellMux/14
  Module14_outputs/7 -> [vParallelAssembly14]
  [vParallelAssembly14] -> vParallelAssemblyMux/14
  Module15_outputs/1 -> [iCell15]
  [iCell15] -> iCellMux/15
  Module15_outputs/2 -> [numCyclesCell15]
  [numCyclesCell15] -> numCyclesCellMux/15
  Module15_outputs/3 -> [socCell15]
  [socCell15] -> socCellMux/15
  Module15_outputs/4 -> [socParallelAssembly15]
  [socParallelAssembly15] -> socParallelAssemblyMux/15
  Module15_outputs/5 -> [temperatureCell15]
  [temperatureCell15] -> temperatureCellMux/15
  Module15_outputs/6 -> [vCell15]
  [vCell15] -> vCellMux/15
  Module15_outputs/7 -> [vParallelAssembly15]
  [vParallelAssembly15] -> vParallelAssemblyMux/15
  Module16_outputs/1 -> [iCell16]
  [iCell16] -> iCellMux/16
  Module16_outputs/2 -> [numCyclesCell16]
  [numCyclesCell16] -> numCyclesCellMux/16
  Module16_outputs/3 -> [socCell16]
  [socCell16] -> socCellMux/16
  Module16_outputs/4 -> [socParallelAssembly16]
  [socParallelAssembly16] -> socParallelAssemblyMux/16
  Module16_outputs/5 -> [temperatureCell16]
  [temperatureCell16] -> temperatureCellMux/16
  Module16_outputs/6 -> [vCell16]
  [vCell16] -> vCellMux/16
  Module16_outputs/7 -> [vParallelAssembly16]
  [vParallelAssembly16] -> vParallelAssemblyMux/16
  Module17_outputs/1 -> [iCell17]
  [iCell17] -> iCellMux/17
  Module17_outputs/2 -> [numCyclesCell17]
  [numCyclesCell17] -> numCyclesCellMux/17
  Module17_outputs/3 -> [socCell17]
  [socCell17] -> socCellMux/17
  Module17_outputs/4 -> [socParallelAssembly17]
  [socParallelAssembly17] -> socParallelAssemblyMux/17
  Module17_outputs/5 -> [temperatureCell17]
  [temperatureCell17] -> temperatureCellMux/17
  Module17_outputs/6 -> [vCell17]
  [vCell17] -> vCellMux/17
  Module17_outputs/7 -> [vParallelAssembly17]
  [vParallelAssembly17] -> vParallelAssemblyMux/17
  Module18_outputs/1 -> [iCell18]
  [iCell18] -> iCellMux/18
  Module18_outputs/2 -> [numCyclesCell18]
  [numCyclesCell18] -> numCyclesCellMux/18
  Module18_outputs/3 -> [socCell18]
  [socCell18] -> socCellMux/18
  Module18_outputs/4 -> [socParallelAssembly18]
  [socParallelAssembly18] -> socParallelAssemblyMux/18
  Module18_outputs/5 -> [temperatureCell18]
  [temperatureCell18] -> temperatureCellMux/18
  Module18_outputs/6 -> [vCell18]
  [vCell18] -> vCellMux/18
  Module18_outputs/7 -> [vParallelAssembly18]
  [vParallelAssembly18] -> vParallelAssemblyMux/18
  Module19_outputs/1 -> [iCell19]
  [iCell19] -> iCellMux/19
  Module19_outputs/2 -> [numCyclesCell19]
  [numCyclesCell19] -> numCyclesCellMux/19
  Module19_outputs/3 -> [socCell19]
  [socCell19] -> socCellMux/19
  Module19_outputs/4 -> [socParallelAssembly19]
  [socParallelAssembly19] -> socParallelAssemblyMux/19
  Module19_outputs/5 -> [temperatureCell19]
  [temperatureCell19] -> temperatureCellMux/19
  Module19_outputs/6 -> [vCell19]
  [vCell19] -> vCellMux/19
  Module19_outputs/7 -> [vParallelAssembly19]
  [vParallelAssembly19] -> vParallelAssemblyMux/19
  Module20_outputs/1 -> [iCell20]
  [iCell20] -> iCellMux/20
  Module20_outputs/2 -> [numCyclesCell20]
  [numCyclesCell20] -> numCyclesCellMux/20
  Module20_outputs/3 -> [socCell20]
  [socCell20] -> socCellMux/20
  Module20_outputs/4 -> [socParallelAssembly20]
  [socParallelAssembly20] -> socParallelAssemblyMux/20
  Module20_outputs/5 -> [temperatureCell20]
  [temperatureCell20] -> temperatureCellMux/20
  Module20_outputs/6 -> [vCell20]
  [vCell20] -> vCellMux/20
  Module20_outputs/7 -> [vParallelAssembly20]
  [vParallelAssembly20] -> vParallelAssemblyMux/20
  Module21_outputs/1 -> [iCell21]
  [iCell21] -> iCellMux/21
  Module21_outputs/2 -> [numCyclesCell21]
  [numCyclesCell21] -> numCyclesCellMux/21
  Module21_outputs/3 -> [socCell21]
  [socCell21] -> socCellMux/21
  Module21_outputs/4 -> [socParallelAssembly21]
  [socParallelAssembly21] -> socParallelAssemblyMux/21
  Module21_outputs/5 -> [temperatureCell21]
  [temperatureCell21] -> temperatureCellMux/21
  Module21_outputs/6 -> [vCell21]
  [vCell21] -> vCellMux/21
  Module21_outputs/7 -> [vParallelAssembly21]
  [vParallelAssembly21] -> vParallelAssemblyMux/21
  Module22_outputs/1 -> [iCell22]
  [iCell22] -> iCellMux/22
  Module22_outputs/2 -> [numCyclesCell22]
  [numCyclesCell22] -> numCyclesCellMux/22
  Module22_outputs/3 -> [socCell22]
  [socCell22] -> socCellMux/22
  Module22_outputs/4 -> [socParallelAssembly22]
  [socParallelAssembly22] -> socParallelAssemblyMux/22
  Module22_outputs/5 -> [temperatureCell22]
  [temperatureCell22] -> temperatureCellMux/22
  Module22_outputs/6 -> [vCell22]
  [vCell22] -> vCellMux/22
  Module22_outputs/7 -> [vParallelAssembly22]
  [vParallelAssembly22] -> vParallelAssemblyMux/22
  Module23_outputs/1 -> [iCell23]
  [iCell23] -> iCellMux/23
  Module23_outputs/2 -> [numCyclesCell23]
  [numCyclesCell23] -> numCyclesCellMux/23
  Module23_outputs/3 -> [socCell23]
  [socCell23] -> socCellMux/23
  Module23_outputs/4 -> [socParallelAssembly23]
  [socParallelAssembly23] -> socParallelAssemblyMux/23
  Module23_outputs/5 -> [temperatureCell23]
  [temperatureCell23] -> temperatureCellMux/23
  Module23_outputs/6 -> [vCell23]
  [vCell23] -> vCellMux/23
  Module23_outputs/7 -> [vParallelAssembly23]
  [vParallelAssembly23] -> vParallelAssemblyMux/23
  Module24_outputs/1 -> [iCell24]
  [iCell24] -> iCellMux/24
  Module24_outputs/2 -> [numCyclesCell24]
  [numCyclesCell24] -> numCyclesCellMux/24
  Module24_outputs/3 -> [socCell24]
  [socCell24] -> socCellMux/24
  Module24_outputs/4 -> [socParallelAssembly24]
  [socParallelAssembly24] -> socParallelAssemblyMux/24
  Module24_outputs/5 -> [temperatureCell24]
  [temperatureCell24] -> temperatureCellMux/24
  Module24_outputs/6 -> [vCell24]
  [vCell24] -> vCellMux/24
  Module24_outputs/7 -> [vParallelAssembly24]
  [vParallelAssembly24] -> vParallelAssemblyMux/24
  Module25_outputs/1 -> [iCell25]
  [iCell25] -> iCellMux/25
  Module25_outputs/2 -> [numCyclesCell25]
  [numCyclesCell25] -> numCyclesCellMux/25
  Module25_outputs/3 -> [socCell25]
  [socCell25] -> socCellMux/25
  Module25_outputs/4 -> [socParallelAssembly25]
  [socParallelAssembly25] -> socParallelAssemblyMux/25
  Module25_outputs/5 -> [temperatureCell25]
  [temperatureCell25] -> temperatureCellMux/25
  Module25_outputs/6 -> [vCell25]
  [vCell25] -> vCellMux/25
  Module25_outputs/7 -> [vParallelAssembly25]
  [vParallelAssembly25] -> vParallelAssemblyMux/25
  Module26_outputs/1 -> [iCell26]
  [iCell26] -> iCellMux/26
  Module26_outputs/2 -> [numCyclesCell26]
  [numCyclesCell26] -> numCyclesCellMux/26
  Module26_outputs/3 -> [socCell26]
  [socCell26] -> socCellMux/26
  Module26_outputs/4 -> [socParallelAssembly26]
  [socParallelAssembly26] -> socParallelAssemblyMux/26
  Module26_outputs/5 -> [temperatureCell26]
  [temperatureCell26] -> temperatureCellMux/26
  Module26_outputs/6 -> [vCell26]
  [vCell26] -> vCellMux/26
  Module26_outputs/7 -> [vParallelAssembly26]
  [vParallelAssembly26] -> vParallelAssemblyMux/26
  Module27_outputs/1 -> [iCell27]
  [iCell27] -> iCellMux/27
  Module27_outputs/2 -> [numCyclesCell27]
  [numCyclesCell27] -> numCyclesCellMux/27
  Module27_outputs/3 -> [socCell27]
  [socCell27] -> socCellMux/27
  Module27_outputs/4 -> [socParallelAssembly27]
  [socParallelAssembly27] -> socParallelAssemblyMux/27
  Module27_outputs/5 -> [temperatureCell27]
  [temperatureCell27] -> temperatureCellMux/27
  Module27_outputs/6 -> [vCell27]
  [vCell27] -> vCellMux/27
  Module27_outputs/7 -> [vParallelAssembly27]
  [vParallelAssembly27] -> vParallelAssemblyMux/27
  connections:
  Module02/LConn1 -- Module01/RConn1
  Module03/LConn1 -- Module02/RConn1
  Module04/LConn1 -- Module03/RConn1
  Module05/LConn1 -- Module04/RConn1
  Module06/LConn1 -- Module05/RConn1
  Module07/LConn1 -- Module06/RConn1
  Module08/LConn1 -- Module07/RConn1
  Module09/LConn1 -- Module08/RConn1
  Module10/LConn1 -- Module09/RConn1
  Module11/LConn1 -- Module10/RConn1
  Module12/LConn1 -- Module11/RConn1
  Module13/LConn1 -- Module12/RConn1
  Module14/LConn1 -- Module13/RConn1
  Module15/LConn1 -- Module14/RConn1
  Module16/LConn1 -- Module15/RConn1
  Module17/LConn1 -- Module16/RConn1
  Module18/LConn1 -- Module17/RConn1
  Module19/LConn1 -- Module18/RConn1
  Module20/LConn1 -- Module19/RConn1
  Module21/LConn1 -- Module20/RConn1
  Module22/LConn1 -- Module21/RConn1
  Module23/LConn1 -- Module22/RConn1
  Module24/LConn1 -- Module23/RConn1
  Module25/LConn1 -- Module24/RConn1
  Module26/LConn1 -- Module25/RConn1
  Module27/LConn1 -- Module26/RConn1
  Module01/LConn1 -- +/RConn1
  Module27/RConn1 -- -/RConn1
